simulink model "systemModel"  (R2018a)
settings: Solver=FixedStepAuto  StartTime=0.0  StopTime=12  FixedStep=0.1  RelTol=1e-3
undefined symbols (not defined in the file): x10, x20
libraries: simulink x1
settings Model: Creator=Martin  LastModifiedBy=Martin

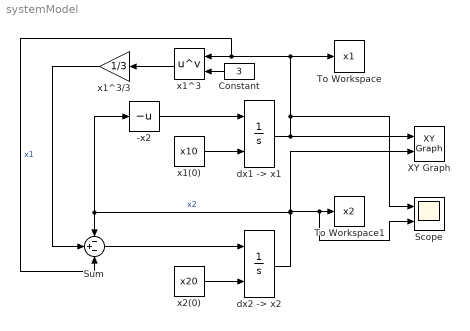
== system systemModel ==
  -x2 : UnaryMinus
  Constant : Constant  Value=3
  Scope : Scope  NumInputPorts=2
  Sum : Sum  Inputs=-+-
  To Workspace : ToWorkspace  VariableName=x1  SaveFormat=Timeseries  SampleTime=-1
  To Workspace1 : ToWorkspace  VariableName=x2  SaveFormat=Timeseries  SampleTime=-1
  XY Graph : simulink/Sinks/XY Graph  xmin=-1  xmax=1  ymin=-1  ymax=1  st=-1
  "dx1 -> x1" : Integrator  InitialConditionSource=external
  "dx2 -> x2" : Integrator  InitialConditionSource=external
  x1(0) : Constant  Value=x10
  x1^3 : Math  Operator=pow  SaturateOnIntegerOverflow=on
  x1^3/3 : Gain  Gain=1/3
  x2(0) : Constant  Value=x20
  wires:
  "dx2 -> x2"/1 -> XY Graph/2, Scope/2, To Workspace1/1, -x2/1, Sum/1  "x2"
  -x2/1 -> "dx1 -> x1"/1
  Sum/1 -> "dx2 -> x2"/1
  "dx1 -> x1"/1 -> XY Graph/1, Scope/1, Sum/3, x1^3/1, To Workspace/1  "x1"
  x1^3/1 -> x1^3/3/1
  x1^3/3/1 -> Sum/2
  x1(0)/1 -> "dx1 -> x1"/2
  x2(0)/1 -> "dx2 -> x2"/2
  Constant/1 -> x1^3/2
